simulink model "Schmitt_Trigger_mod_e"  (R2020b)
settings: Solver=FixedStepAuto  StartTime=0.0  StopTime=2/20  FixedStep=1/2000  RelTol=1e-3
values from neighbouring files (symbols this model uses):
  A = 5    [Schmitt_Trigger_data_a.m]    (also in UE2_1.m = 3; UE5_1.m = 3; Wdh4_1_RauschsignalGenerieren.m = 0.4)
  f = (0:N)*f0    [SUT.m]    (also in Schmitt_Trigger_data_a.m = 20; UE1_3.m = repelem(e,5); UE6_1.m; Wdh1_3_Signalvektoren.m = [e e e e e])
  Ua = 5    [Schmitt_Trigger_data_a.m]
  Us = 1    [Schmitt_Trigger_data_a.m]
settings Model: Creator=Sinh  LastModifiedBy=Sinh

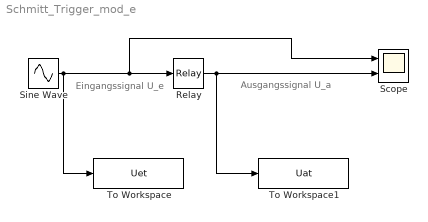
== system Schmitt_Trigger_mod_e ==
  note: Ausgangssignal U_a
  note: Eingangssignal U_e
  Relay : Relay  OnSwitchValue=Us  OffSwitchValue=-Us  OnOutputValue=Ua  OffOutputValue=-Ua
  Scope : Scope  NumInputPorts=2
  Sine Wave : Sin  Amplitude=A  Frequency=2*pi*f  SampleTime=0
  To Workspace : ToWorkspace  VariableName=Uet  SampleTime=-1
  To Workspace1 : ToWorkspace  VariableName=Uat  SampleTime=-1
  wires:
  Sine Wave/1 -> To Workspace/1, Scope/1, Relay/1
  Relay/1 -> To Workspace1/1, Scope/2
